simulink model "GOcontrollProject"  (R2023b)
settings: Solver=FixedStepDiscrete  StartTime=0.0  StopTime=5  FixedStep=0.01  RelTol=1e-3
PostLoadFcn:
  | try
  |     eval([bdroot,'_startup']) %to run model_startup.m
  | catch
  |     disp("No startup file found for this model");
  | end
  | core_info = evalc('feature(''numcores'')');
  | core_info_split = split(core_info, " ");
  | num_cores = core_info_split{12};
  | set_param(bdroot, "MakeCommand", ['make_rtw -j' num_cores]);
  | clear num_cores core_info core_info_split
libraries: GOcontroll_Moduline_Target x9
settings Model: Creator=DeveloperGOcontroll  LastModifiedBy=DeveloperGOcontroll
settings SolverCC: AlgebraicLoopSolver=TrustRegion
settings DataIOCC: LimitDataPoints=on  SaveFormat=Array  ReturnWorkspaceOutputs=off
settings OptimizationCC: BlockReduction=off  DefaultParameterBehavior=Inlined  EnhancedBackFolding=on  PassReuseOutputArgsAs=Individual arguments  ZeroExternalMemoryAtStartup=off  ZeroInternalMemoryAtStartup=off  OptimizeBlockOrder=speed  DifferentSizesBufferReuse=on  OptimizationCustomize=off  EfficientTunableParamExpr=on
settings DebuggingCC: SolverPrmCheckMsg=warning  InheritedTsInSrcMsg=none  MultiTaskRateTransMsg=warning  ParameterPrecisionLossMsg=none  ParameterTunabilityLossMsg=error  UnconnectedInputMsg=error  UnconnectedOutputMsg=error  UnconnectedLineMsg=error  SFUnusedDataAndEventsDiag=none  SFUnexpectedBacktrackingDiag=warning  SFNoUnconditionalDefaultTransitionDiag=warning  SFUndirectedBroadcastEventsDiag=none  SFExecutionAtInitializationDiag=none  RCSCRenamedMsg=none  RCSCObservableMsg=none  ArithmeticOperatorsInVariantConditions=warning
settings HardwareCC: ProdBitPerPointer=32  ProdBitPerSizeT=32  ProdBitPerPtrDiffT=32  ProdLargestAtomicInteger=Long  ProdLargestAtomicFloat=Double  ProdWordSize=32  ProdHWDeviceType=ARM Compatible->ARM Cortex-M
settings ModelReferenceCC: EnableRefExpFcnMdlSchedulingChecks=on  PropagateSignalLabelsOutOfModel=off
settings SFSimCC: SimUseLocalCustomCode=off  MATLABDynamicMemAlloc=off  CustomCodeUndefinedFunction=UseInterfaceOnly
settings RTWCC: Description=GOcontroll Embedded Coder  SystemTargetFile=ert_linux.tlc  MakeCommand=make_rtw -j32  TemplateMakefile=ert_linux_target_64.tmf  RetainRTWFile=on  RTWUseLocalCustomCode=off
settings CodeAppCC: ForceParamTrailComments=on  IgnoreCustomStorageClasses=off  OperatorAnnotations=on  SimulinkDataObjDesc=on  SFDataObjDesc=on  InsertBlockDesc=on
settings STFCustomTargetCC: TargetLangStandard=C89/C90 (ANSI)  MultiwordLength=256  CombineOutputUpdateFcns=on  ERTCustomFileBanners=on  SupportContinuousTime=off  SupportNonInlinedSFcns=off  RemoveResetFunc=on  MATLABClassNameForMDSCustomization=Simulink.SoftwareTarget.ERTCustomization  SystemTargetFile=ert_linux.tlc
settings ERTTargetCC: ParMdlRefBuildCompliant=off  CompOptLevelCompliant=off  ConcurrentExecutionCompliant=off  ModelStepFunctionPrototypeControlCompliant=off  CPPClassGenCompliant=off  UseToolchainInfoCompliant=off  InlinedParameterPlacement=NonHierarchical  ERTCustomFileTemplate=ert_linux_file_process.tlc
settings ConfigComp: CovMetricSettings=dw  CovSaveCumulativeToWorkspaceVar=on  CovSaveSingleToWorkspaceVar=on  CovExternalEMLEnable=off  CovSFcnEnable=off

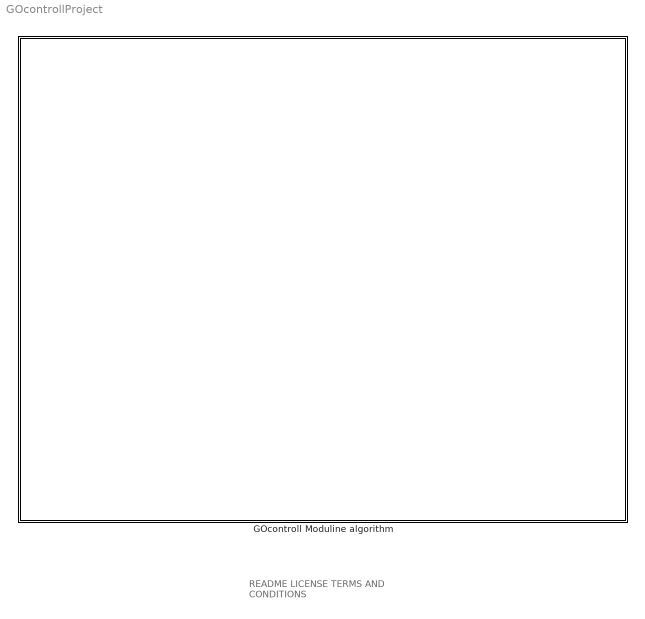
== system GOcontrollProject ==
  note: README
      |
      | LICENSE
      |
      | TERMS AND CONDITIONS
  GOcontroll Moduline algorithm : Subsystem  mask(TopLevelSubsystem){}
      mask Display: image(gocontroll_png())

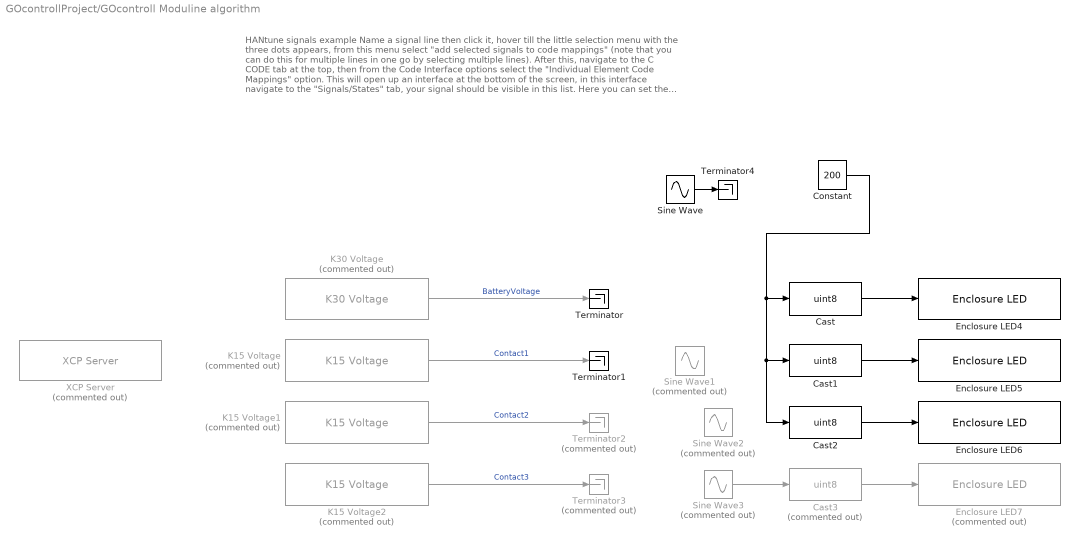
== system GOcontrollProject/GOcontroll Moduline algorithm ==
  note: HANtune signals example
      | Name a signal line then click it, hover till the little selection menu with
      | the three dots appears, from this menu select "add selected signals
      | to code mappings" (note that you can do this for multiple lines in one go
      | by selecting multiple lines).
      | After this, navigate to the C CODE tab at the top, then from the Code
      | Interface options select the "Individual Element Code Mappings" option.
      | This will open up an interface at the bottom of the screen, in this interface
      | navigate to the "Signals/States" tab, your signal should be visible in this list.
      | Here you can set the storage class to "ExportedGlobal", this can also be
      | done for multiple signals in one go by selecting multiple signals in the list
      | with ctrl or shift click, and then changing the storage class for any of the
      | selected signals.
  Cast : DataTypeConversion  OutDataTypeStr=uint8  SaturateOnIntegerOverflow=off  RndMeth=Floor
  Cast1 : DataTypeConversion  OutDataTypeStr=uint8  SaturateOnIntegerOverflow=off  RndMeth=Floor
  Cast2 : DataTypeConversion  OutDataTypeStr=uint8  SaturateOnIntegerOverflow=off  RndMeth=Floor
  Cast3 : DataTypeConversion  Commented=on  OutDataTypeStr=uint8  SaturateOnIntegerOverflow=off  RndMeth=Floor
  Constant : Constant  Value=200
  Enclosure LED4 : GOcontroll_Moduline_Target/Enclosure LED's/Enclosure LED  Tag=HANcoder_GOcontroll_Moduline_IV  tsamp=1  led=1  color=Red
      settings: SourceProductName=GOcontroll Moduline
  Enclosure LED5 : GOcontroll_Moduline_Target/Enclosure LED's/Enclosure LED  Tag=HANcoder_GOcontroll_Moduline_IV  tsamp=1  led=1  color=Blue
      settings: SourceProductName=GOcontroll Moduline
  Enclosure LED6 : GOcontroll_Moduline_Target/Enclosure LED's/Enclosure LED  Tag=HANcoder_GOcontroll_Moduline_IV  tsamp=1  led=1  color=Green
      settings: SourceProductName=GOcontroll Moduline
  Enclosure LED7 : GOcontroll_Moduline_Target/Enclosure LED's/Enclosure LED  Tag=HANcoder_GOcontroll_Moduline_IV  Commented=on  tsamp=-1  led=4  color=Blue
      settings: SourceProductName=GOcontroll Moduline
  K15 Voltage : GOcontroll_Moduline_Target/Supply control/K15 Voltage  Tag=HANcoder_GOcontroll_Moduline_IV  Commented=on  ContrType=GOcontroll Moduline IV  tsamp=0.1  k15pin=K15-1 (Connector C pin 2)
      settings: SourceProductName=GOcontroll Moduline
  K15 Voltage1 : GOcontroll_Moduline_Target/Supply control/K15 Voltage  Tag=HANcoder_GOcontroll_Moduline_IV  Commented=on  ContrType=GOcontroll Moduline IV  tsamp=0.1  k15pin=K15-2 (Connector C pin 3)
      settings: SourceProductName=GOcontroll Moduline
  K15 Voltage2 : GOcontroll_Moduline_Target/Supply control/K15 Voltage  Tag=HANcoder_GOcontroll_Moduline_IV  Commented=on  ContrType=GOcontroll Moduline IV  tsamp=0.1  k15pin=K15-3 (Connector C pin 4)
      settings: SourceProductName=GOcontroll Moduline
  K30 Voltage : GOcontroll_Moduline_Target/Supply control/K30 Voltage  Tag=HANcoder_GOcontroll_Moduline_IV  Commented=on  ContrType=GOcontroll Moduline IV  tsamp=0.1
      settings: SourceProductName=GOcontroll Moduline
  Sine Wave : Sin  SineType=Sample based  Amplitude=120  Bias=120  Samples=200  SampleTime=0.01
  Sine Wave1 : Sin  Commented=on  SineType=Sample based  Amplitude=75  Bias=75  Samples=200  SampleTime=0.01  Offset=50
  Sine Wave2 : Sin  Commented=on  SineType=Sample based  Amplitude=75  Bias=75  Samples=200  SampleTime=0.01  Offset=100
  Sine Wave3 : Sin  Commented=on  SineType=Sample based  Amplitude=75  Bias=75  Samples=200  SampleTime=0.01  Offset=150
  Terminator : Terminator
  Terminator1 : Terminator
  Terminator2 : Terminator  Commented=on
  Terminator3 : Terminator  Commented=on
  Terminator4 : Terminator
  XCP Server : GOcontroll_Moduline_Target/System/XCP Server  Priority=999999  Commented=on  ContrType=GOcontroll Moduline IV  server_type=TCP  can_if=CAN1 - Connector C pin 14 (L) and pin 15 (H)  receive_id=hex2dec('665')  send_id=hex2dec('666')
      settings: SourceProductName=GOcontroll Moduline
  wires:
  K15 Voltage/1 -> Terminator1/1  "Contact1"
  K15 Voltage2/1 -> Terminator3/1  "Contact3"
  K30 Voltage/1 -> Terminator/1  "BatteryVoltage"
  K15 Voltage1/1 -> Terminator2/1  "Contact2"
  Sine Wave/1 -> Terminator4/1
  Cast1/1 -> Enclosure LED5/1
  Cast3/1 -> Enclosure LED7/1
  Sine Wave3/1 -> Cast3/1
  Cast2/1 -> Enclosure LED6/1
  Constant/1 -> Cast2/1, Cast1/1, Cast/1
  Cast/1 -> Enclosure LED4/1
